simulink model "quiz"  (R2015a)
settings: Solver=ode45  StartTime=0.0  StopTime=10.0  RelTol=1e-3
undefined symbols (not defined in the file): b, k, m
settings Model: Creator=eric  LastModifiedBy=eric

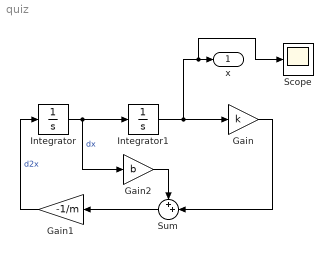
== system quiz ==
  Gain : Gain  Gain=k
  Gain1 : Gain  Gain=-1/m
  Gain2 : Gain  Gain=b
  Integrator : Integrator  InitialCondition=10
  Integrator1 : Integrator
  Scope : Scope
  Sum : Sum  Inputs=++|
  x : Outport
  wires:
  Integrator/1 -> Gain2/1, Integrator1/1  "dx"
  Integrator1/1 -> Gain/1, x/1, Scope/1
  Gain1/1 -> Integrator/1  "d2x"
  Sum/1 -> Gain1/1
  Gain/1 -> Sum/2
  Gain2/1 -> Sum/1
